simulink model "Task2PI"  (R2022a)
settings: Solver=FixedStepAuto  StartTime=0.0  StopTime=100  FixedStep=0.001  RelTol=1e-3
undefined symbols (not defined in the file): k_avg, ki, kp, Tm_avg
settings Model: Creator=Family  LastModifiedBy=Family

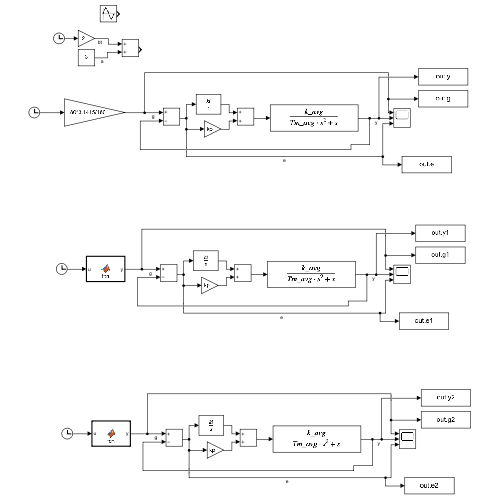
[thumbnail: Simulink's stored preview of the top-level diagram]
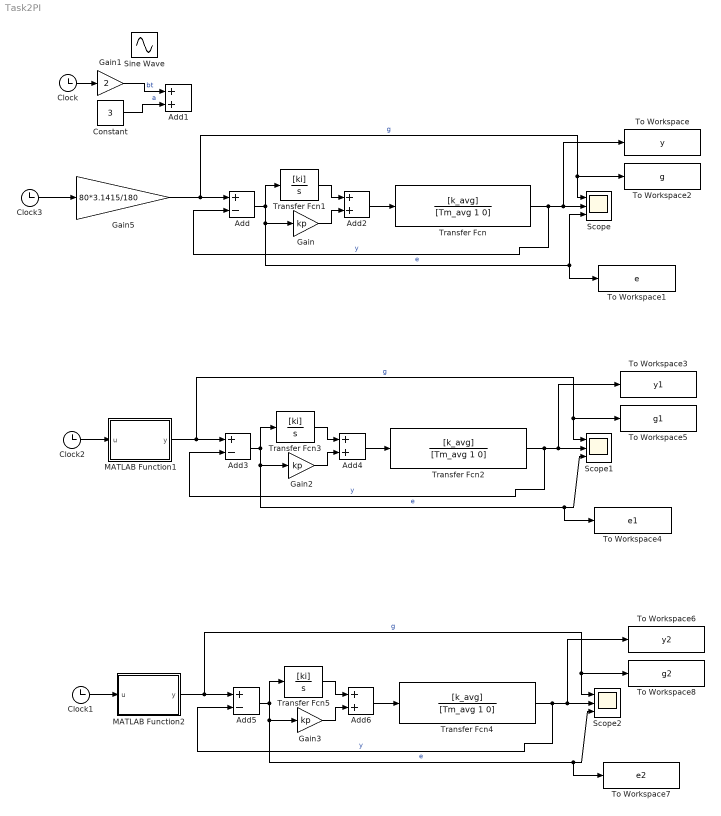
== system Task2PI ==
  Add : Sum  Inputs=+-
  Add{1..2,4,6} (4 alike) : Sum
  Add3 : Sum  Inputs=+-
  Add5 : Sum  Inputs=+-
  Clock{,1..3} (4 alike) : Clock
  Constant : Constant  Value=3
  Gain : Gain  Gain=kp
  Gain1 : Gain  Gain=2
  Gain2 : Gain  Gain=kp
  Gain3 : Gain  Gain=kp
  Gain5 : Gain  Gain=80*3.1415/180
  MATLAB Function1 : MATLAB Function  TreatAsAtomicUnit=on
  MATLAB Function2 : MATLAB Function  TreatAsAtomicUnit=on
  Scope : Scope  NumInputPorts=3
  Scope1 : Scope  NumInputPorts=3
  Scope2 : Scope  NumInputPorts=3
  Sine Wave : Sin  Amplitude=2  Phase=2  SampleTime=0
  To Workspace : ToWorkspace  VariableName=y  SaveFormat=Timeseries  SampleTime=-1
  To Workspace1 : ToWorkspace  VariableName=e  SaveFormat=Timeseries  SampleTime=-1
  To Workspace2 : ToWorkspace  VariableName=g  SaveFormat=Timeseries  SampleTime=-1
  To Workspace3 : ToWorkspace  VariableName=y1  SaveFormat=Timeseries  SampleTime=-1
  To Workspace4 : ToWorkspace  VariableName=e1  SaveFormat=Timeseries  SampleTime=-1
  To Workspace5 : ToWorkspace  VariableName=g1  SaveFormat=Timeseries  SampleTime=-1
  To Workspace6 : ToWorkspace  VariableName=y2  SaveFormat=Timeseries  SampleTime=-1
  To Workspace7 : ToWorkspace  VariableName=e2  SaveFormat=Timeseries  SampleTime=-1
  To Workspace8 : ToWorkspace  VariableName=g2  SaveFormat=Timeseries  SampleTime=-1
  Transfer Fcn : TransferFcn  Numerator=[k_avg]  Denominator=[Tm_avg 1 0]
  Transfer Fcn1 : TransferFcn  Numerator=[ki]  Denominator=[1 0]
  Transfer Fcn2 : TransferFcn  Numerator=[k_avg]  Denominator=[Tm_avg 1 0]
  Transfer Fcn3 : TransferFcn  Numerator=[ki]  Denominator=[1 0]
  Transfer Fcn4 : TransferFcn  Numerator=[k_avg]  Denominator=[Tm_avg 1 0]
  Transfer Fcn5 : TransferFcn  Numerator=[ki]  Denominator=[1 0]
  wires:
  Transfer Fcn/1 -> To Workspace/1, Scope/2, Add/2  "y"
  Add/1 -> To Workspace1/1, Scope/3, Gain/1, Transfer Fcn1/1  "e"
  Gain5/1 -> Add/1, To Workspace2/1, Scope/1  "g"
  Add2/1 -> Transfer Fcn/1
  Clock/1 -> Gain1/1
  Gain1/1 -> Add1/1  "bt"
  Constant/1 -> Add1/2  "a"
  Gain/1 -> Add2/2
  Transfer Fcn1/1 -> Add2/1
  Clock2/1 -> MATLAB Function1/1(u)
  Gain2/1 -> Add4/2
  Add4/1 -> Transfer Fcn2/1
  MATLAB Function1/1(y) -> Add3/1, To Workspace5/1, Scope1/1  "g"
  Transfer Fcn3/1 -> Add4/1
  Add3/1 -> To Workspace4/1, Scope1/3, Gain2/1, Transfer Fcn3/1  "e"
  Transfer Fcn2/1 -> To Workspace3/1, Scope1/2, Add3/2  "y"
  Clock3/1 -> Gain5/1
  Transfer Fcn4/1 -> To Workspace6/1, Scope2/2, Add5/2  "y"
  Add5/1 -> To Workspace7/1, Scope2/3, Gain3/1, Transfer Fcn5/1  "e"
  Transfer Fcn5/1 -> Add6/1
  MATLAB Function2/1(y) -> Add5/1, To Workspace8/1, Scope2/1  "g"
  Clock1/1 -> MATLAB Function2/1(u)
  Add6/1 -> Transfer Fcn4/1
  Gain3/1 -> Add6/2

== matlab function Task2PI/MATLAB Function2 ==
  data: u input; y output
function y = fcn(u)

y = 10*3.14/180*u*u*u;

== matlab function Task2PI/MATLAB Function1 ==
  data: u input; y output
function y = fcn(u)

y = 40*3.1415/180*u*u;
